simulink model "Effectors_UltraStick25e"  (R2016b)
settings: Solver=VariableStepAuto  StartTime=0.0  StopTime=10  FixedStep=SampleTime  RelTol=1e-3
undefined symbols (not defined in the file): AC, Sim
libraries: SurfLib x6
settings Model: Creator=Paul Freeman  LastModifiedBy=rega0051
settings DataIOCC: SaveOutput=off  SignalLogging=off  DSMLogging=off  SaveTime=off
settings OptimizationCC: ExpressionDepthLimit=2147483647  LifeSpan=inf
settings DebuggingCC: SignalInfNanChecking=warning  SaveWithParameterizedLinksMsg=none  UnderspecifiedInitializationDetection=Classic  MergeDetectMultiDrivingBlocksExec=none  CheckMatrixSingularityMsg=warning  UnnecessaryDatatypeConvMsg=warning  FcnCallInpInsideContextMsg=warning  UnconnectedInputMsg=none  UnconnectedOutputMsg=none  UnconnectedLineMsg=none  SFcnCompatibilityMsg=warning  UniqueDataStoreMsg=warning  StateNameClashWarn=warning  StrictBusMsg=WarnOnBusTreatedAsVector  SFUnexpectedBacktrackingDiag=warning  SFNoUnconditionalDefaultTransitionDiag=warning  SFExecutionAtInitializationDiag=none
settings HardwareCC: ProdBitPerPointer=32  ProdBitPerSizeT=32  ProdBitPerPtrDiffT=32  ProdLargestAtomicFloat=None  ProdWordSize=32  ProdHWDeviceType=Custom Processor->Custom
settings GRTTargetCC: TargetLangStandard=C89/C90 (ANSI)  GeneratePreprocessorConditionals=Disable all  CombineOutputUpdateFcns=off  GRTInterface=on
settings ConfigComp: CovMetricSettings=dw  CovHtmlReporting=on  CovSaveCumulativeToWorkspaceVar=on  CovSaveSingleToWorkspaceVar=on  CovExternalEMLEnable=off  CovSFcnEnable=off

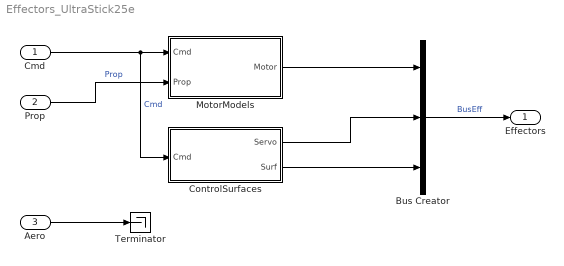
== system Effectors_UltraStick25e ==
  Cmd : Inport  OutDataTypeStr=Bus: BusCmd  SampleTime=0
      settings: AttributesFormatString=%<OutDataTypeStr>
  Prop : Inport  Port=2  OutDataTypeStr=Bus: BusProp  SampleTime=0
      settings: AttributesFormatString=%<OutDataTypeStr>
  Aero : Inport  Port=3  OutDataTypeStr=Bus: BusAero  SampleTime=0
      settings: AttributesFormatString=%<OutDataTypeStr>
  Bus Creator : BusCreator  Inputs=3  OutDataTypeStr=Bus: BusEff
      settings: AttributesFormatString=%<OutDataTypeStr>  InheritFromInputs=off
  ControlSurfaces : Subsystem
  MotorModels : Subsystem
  Terminator : Terminator
  Effectors : Outport  OutDataTypeStr=Bus: BusEff  SampleTime=0
      settings: AttributesFormatString=%<OutDataTypeStr>
  wires:
  ControlSurfaces/1(Servo) -> Bus Creator/2
  MotorModels/1(Motor) -> Bus Creator/1
  Cmd/1 -> ControlSurfaces/1(Cmd), MotorModels/1(Cmd)  "Cmd"
  ControlSurfaces/2(Surf) -> Bus Creator/3
  Bus Creator/1 -> Effectors/1  "BusEff"
  Prop/1 -> MotorModels/2(Prop)  "Prop"
  Aero/1 -> Terminator/1

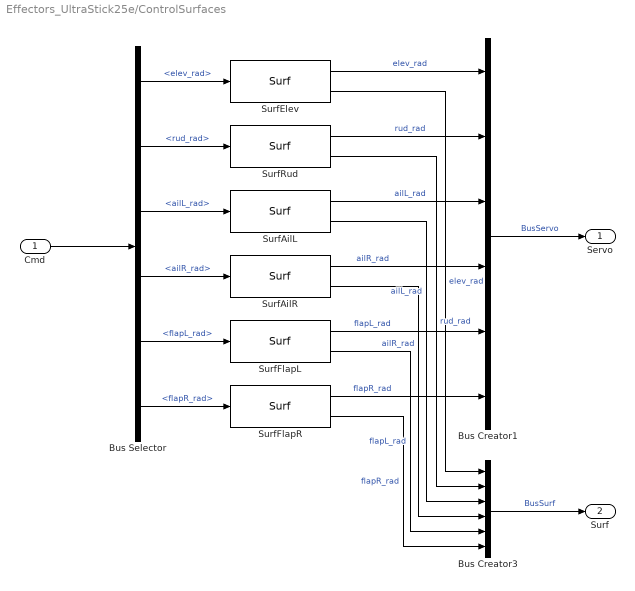
== system Effectors_UltraStick25e/ControlSurfaces ==
  Cmd : Inport
  Bus Creator1 : BusCreator  Inputs=6  OutDataTypeStr=Bus: BusServo
      settings: AttributesFormatString=%<OutDataTypeStr>  InheritFromInputs=off
  Bus Creator3 : BusCreator  Inputs=6  OutDataTypeStr=Bus: BusSurf
      settings: AttributesFormatString=%<OutDataTypeStr>  InheritFromInputs=off
  Bus Selector : BusSelector  OutputSignals=elev_rad,rud_rad,ailL_rad,ailR_rad,flapL_rad,flapR_rad
  SurfAilL : SurfLib/Surf  SurfName='ailL'  SurfParam=AC.Surf.ailL  Init=Sim.Trim.Init
  SurfAilR : SurfLib/Surf  SurfName='ailR'  SurfParam=AC.Surf.ailR  Init=Sim.Trim.Init
  SurfElev : SurfLib/Surf  SurfName='elev'  SurfParam=AC.Surf.elev  Init=Sim.Trim.Init
  SurfFlapL : SurfLib/Surf  SurfName='flapL'  SurfParam=AC.Surf.flapL  Init=Sim.Trim.Init
  SurfFlapR : SurfLib/Surf  SurfName='flapR'  SurfParam=AC.Surf.flapR  Init=Sim.Trim.Init
  SurfRud : SurfLib/Surf  SurfName='rud'  SurfParam=AC.Surf.rud  Init=Sim.Trim.Init
  Servo : Outport
  Surf : Outport  Port=2
  wires:
  SurfElev/1 -> Bus Creator1/1  "elev_rad"
  Bus Creator3/1 -> Surf/1  "BusSurf"
  SurfFlapR/2 -> Bus Creator3/6  "flapR_rad"
  SurfFlapL/2 -> Bus Creator3/5  "flapL_rad"
  SurfAilR/2 -> Bus Creator3/4  "ailR_rad"
  SurfAilL/2 -> Bus Creator3/3  "ailL_rad"
  SurfRud/2 -> Bus Creator3/2  "rud_rad"
  SurfElev/2 -> Bus Creator3/1  "elev_rad"
  Bus Selector/4 -> SurfAilR/1  "<ailR_rad>"
  SurfRud/1 -> Bus Creator1/2  "rud_rad"
  Bus Selector/6 -> SurfFlapR/1  "<flapR_rad>"
  SurfFlapR/1 -> Bus Creator1/6  "flapR_rad"
  SurfAilR/1 -> Bus Creator1/4  "ailR_rad"
  SurfFlapL/1 -> Bus Creator1/5  "flapL_rad"
  Bus Selector/5 -> SurfFlapL/1  "<flapL_rad>"
  SurfAilL/1 -> Bus Creator1/3  "ailL_rad"
  Bus Selector/3 -> SurfAilL/1  "<ailL_rad>"
  Bus Selector/2 -> SurfRud/1  "<rud_rad>"
  Bus Selector/1 -> SurfElev/1  "<elev_rad>"
  Cmd/1 -> Bus Selector/1
  Bus Creator1/1 -> Servo/1  "BusServo"

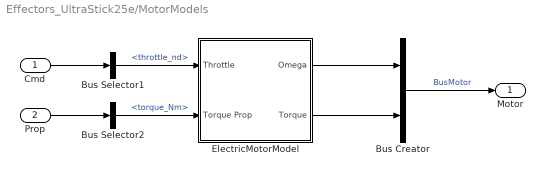
== system Effectors_UltraStick25e/MotorModels ==
  Cmd : Inport  OutDataTypeStr=double
  Prop : Inport  Port=2  OutDataTypeStr=double
  Bus Creator : BusCreator  Inputs=2  OutDataTypeStr=Bus: BusMotor
      settings: AttributesFormatString=%<OutDataTypeStr>  InheritFromInputs=off
  Bus Selector1 : BusSelector  OutputSignals=throttle_nd
  Bus Selector2 : BusSelector  OutputSignals=torque_Nm
  ElectricMotorModel : Subsystem  mask{MotorParam=AC.Motor, Init=Sim.Trim.Init}
      mask prompts: MotorParam "Motor Parameter Structure:"; Init "Motor Initialization Stucture:"
  Motor : Outport
  wires:
  Bus Creator/1 -> Motor/1  "BusMotor"
  Cmd/1 -> Bus Selector1/1
  Bus Selector1/1 -> ElectricMotorModel/1(Throttle)  "<throttle_nd>"
  Bus Selector2/1 -> ElectricMotorModel/2(Torque Prop)  "<torque_Nm>"
  Prop/1 -> Bus Selector2/1
  ElectricMotorModel/1(Omega) -> Bus Creator/1
  ElectricMotorModel/2(Torque) -> Bus Creator/2

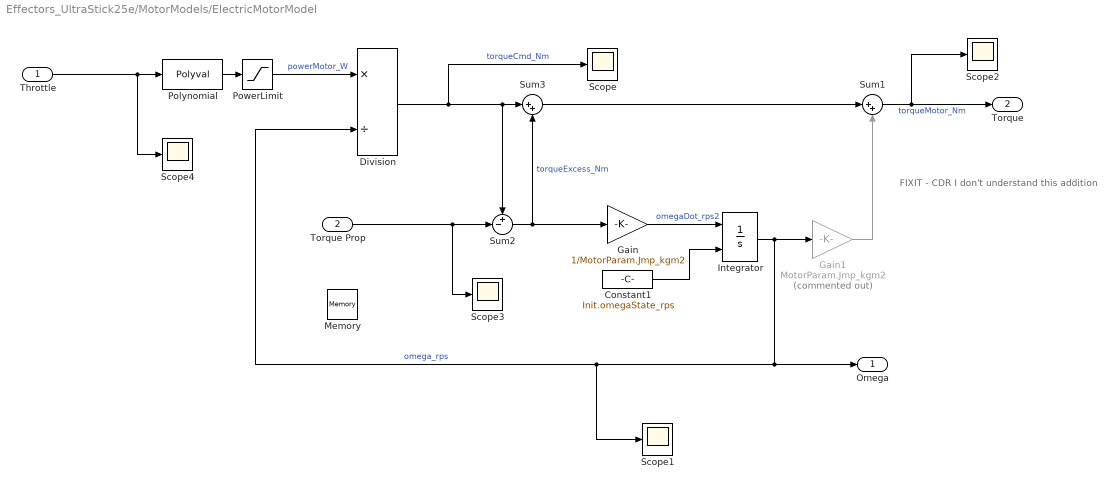
== system Effectors_UltraStick25e/MotorModels/ElectricMotorModel ==
  note: FIXIT - CDR I don't understand this addition
  Throttle : Inport
  Torque Prop : Inport  Port=2
  Constant1 : Constant  Value=Init.omegaState_rps
      settings: AttributesFormatString=%<Value>
  Division : Product  Inputs=*/  SaturateOnIntegerOverflow=on  InputSameDT=on  OutDataTypeStr=Inherit: Same as first input
  Gain : Gain  Gain=1/MotorParam.Jmp_kgm2
      settings: AttributesFormatString=%<Gain>
  Gain1 : Gain  Commented=on  Gain=MotorParam.Jmp_kgm2
      settings: AttributesFormatString=%<Gain>
  Integrator : Integrator  InitialConditionSource=external  LimitOutput=on  UpperSaturationLimit=MotorParam.omegaLimPos_rps  LowerSaturationLimit=MotorParam.omegaLimNeg_rps  ContinuousStateAttributes='omegaState_rps'
      settings: AttributesFormatString=State: %<ContinuousStateAttributes>
  Memory : Memory
  Polynomial : Polyval  Coefs=MotorParam.power_w
  PowerLimit : Saturate  UpperLimit=MotorParam.powerLimPos_w  LowerLimit=MotorParam.powerLimNeg_w
  Scope{,1..4} (5 alike) : Scope
  Sum1 : Sum  Inputs=|++  SaturateOnIntegerOverflow=on
  Sum2 : Sum  Inputs=+-|  SaturateOnIntegerOverflow=on
  Sum3 : Sum  Inputs=|++  SaturateOnIntegerOverflow=on
  Omega : Outport
  Torque : Outport  Port=2
  wires:
  Throttle/1 -> Scope4/1, Polynomial/1
  Constant1/1 -> Integrator/2
  Gain/1 -> Integrator/1  "omegaDot_rps2"
  Sum2/1 -> Gain/1, Sum3/2  "torqueExcess_Nm"
  Integrator/1 -> Gain1/1, Scope1/1, Division/2, Omega/1  "omega_rps"
  Sum3/1 -> Sum1/1
  Polynomial/1 -> PowerLimit/1
  Division/1 -> Scope/1, Sum2/1, Sum3/1  "torqueCmd_Nm"
  Torque Prop/1 -> Scope3/1, Sum2/2
  PowerLimit/1 -> Division/1  "powerMotor_W"
  Sum1/1 -> Scope2/1, Torque/1  "torqueMotor_Nm"
  Gain1/1 -> Sum1/2
